simulink model "train_set"  (R2021a)
settings: Solver=VariableStepAuto  StartTime=0.0  StopTime=100  RelTol=1e-3
libraries: simulink x3
settings Model: Creator=hty  LastModifiedBy=hty

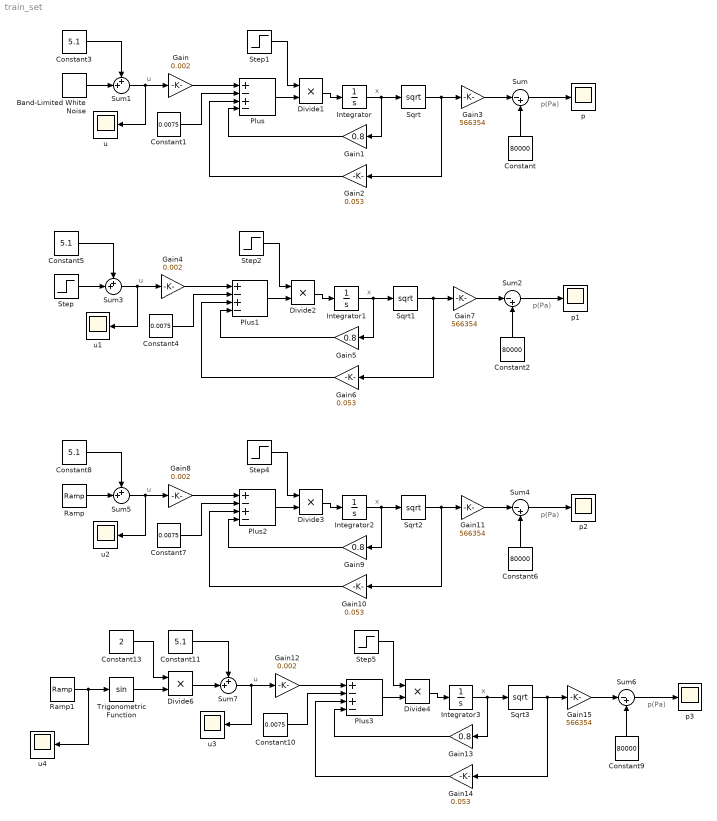
== system train_set ==
  note: p(Pa)
  note: u
  note: x
  note: x
  note: u
  note: p(Pa)
  note: p(Pa)
  note: u
  note: x
  note: p(Pa)
  note: u
  note: x
  Band-Limited White Noise : simulink/Sources/Band-Limited White Noise  Cov=[0.1]  Ts=0.01  seed=[23341]
  Constant{,2,6,9} (4 alike) : Constant  Value=80000
  Constant{1,4,7,10} (4 alike) : Constant  Value=0.0075
  Constant{3,5,8,11} (4 alike) : Constant  Value=5.1
  Constant13 : Constant  Value=2
  Divide{1..4,6} (5 alike) : Product  Inputs=**
  Gain{,4,8,12} (4 alike) : Gain  Gain=0.002
  Gain{1,5,9,13} (4 alike) : Gain  Gain=0.8
  Gain{2,6,10,14} (4 alike) : Gain  Gain=0.053
  Gain{3,7,11,15} (4 alike) : Gain  Gain=566354
  Integrator{,1..3} (4 alike) : Integrator  InitialCondition=0.01
  Plus{,1..3} (4 alike) : Sum  Inputs=+-+-
  Ramp : simulink/Sources/Ramp  slope=0.01  start=0  InitialOutput=0
  Ramp1 : simulink/Sources/Ramp  slope=5  start=0  InitialOutput=0
  Sqrt{,1..3} (4 alike) : Sqrt  SaturateOnIntegerOverflow=on
  Step : Step  Time=0  After=0.51  SampleTime=0.01
  Step{1..2,4..5} (4 alike) : Step  Time=0  SampleTime=0
  Sum{,2,4,6} (4 alike) : Sum  Inputs=|-+
  Sum{1,3,5,7} (4 alike) : Sum  Inputs=++|
  Trigonometric Function : Trigonometry
  p{,1..3} (4 alike) : Scope
  u{,1..4} (5 alike) : Scope
  wires:
  Gain/1 -> Plus/1
  Integrator/1 -> Gain1/1, Sqrt/1
  Gain1/1 -> Plus/4
  Sqrt/1 -> Gain2/1, Gain3/1
  Gain3/1 -> Sum/1
  Constant/1 -> Sum/2
  Gain2/1 -> Plus/3
  Constant1/1 -> Plus/2
  Plus/1 -> Divide1/2
  Step1/1 -> Divide1/1
  Divide1/1 -> Integrator/1
  Band-Limited White Noise/1 -> Sum1/2
  Sum1/1 -> Gain/1, u/1
  Constant3/1 -> Sum1/1
  Sum/1 -> p/1
  Gain5/1 -> Plus1/4
  Constant2/1 -> Sum2/2
  Gain4/1 -> Plus1/1
  Constant4/1 -> Plus1/2
  Plus1/1 -> Divide2/2
  Integrator1/1 -> Gain5/1, Sqrt1/1
  Divide2/1 -> Integrator1/1
  Sum3/1 -> Gain4/1, u1/1
  Sqrt1/1 -> Gain6/1, Gain7/1
  Gain7/1 -> Sum2/1
  Gain6/1 -> Plus1/3
  Sum2/1 -> p1/1
  Step2/1 -> Divide2/1
  Step/1 -> Sum3/2
  Constant5/1 -> Sum3/1
  Sum5/1 -> Gain8/1, u2/1
  Constant6/1 -> Sum4/2
  Integrator2/1 -> Gain9/1, Sqrt2/1
  Constant8/1 -> Sum5/1
  Divide3/1 -> Integrator2/1
  Step4/1 -> Divide3/1
  Plus2/1 -> Divide3/2
  Sqrt2/1 -> Gain10/1, Gain11/1
  Ramp/1 -> Sum5/2
  Constant7/1 -> Plus2/2
  Gain9/1 -> Plus2/4
  Gain11/1 -> Sum4/1
  Gain8/1 -> Plus2/1
  Sum4/1 -> p2/1
  Gain10/1 -> Plus2/3
  Sum7/1 -> Gain12/1, u3/1
  Constant9/1 -> Sum6/2
  Integrator3/1 -> Gain13/1, Sqrt3/1
  Constant11/1 -> Sum7/1
  Divide4/1 -> Integrator3/1
  Step5/1 -> Divide4/1
  Plus3/1 -> Divide4/2
  Sqrt3/1 -> Gain14/1, Gain15/1
  Constant10/1 -> Plus3/2
  Gain13/1 -> Plus3/4
  Gain15/1 -> Sum6/1
  Gain12/1 -> Plus3/1
  Sum6/1 -> p3/1
  Gain14/1 -> Plus3/3
  Ramp1/1 -> u4/1, Trigonometric Function/1
  Divide6/1 -> Sum7/2
  Constant13/1 -> Divide6/1
  Trigonometric Function/1 -> Divide6/2
